simulink model "Preleva2"  (R2019a)
settings: Solver=VariableStepAuto  StartTime=0.0  StopTime=10.0  RelTol=1e-3
settings Model: Creator=anton  LastModifiedBy=anton

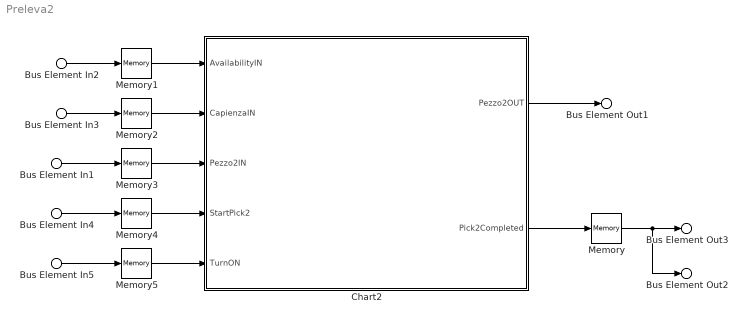
== system Preleva2 ==
  Bus Element In2 : Inport  PortName=Availability2IN
  Bus Element In3 : Inport  Port=2  PortName=Capienza2IN
  Bus Element In4 : Inport  Port=3  PortName=StartPick2
  Bus Element In5 : Inport  Port=4  PortName=TurnON
  Bus Element In1 : Inport  Port=5  PortName=Pezzo2
  Chart2 : Stateflow chart  BlockKeywords=__PRM__SERIALIZED__DATA__:Stateflow Chart,Stateflow Diagram  TreatAsAtomicUnit=on
  Memory{,1..5} (6 alike) : Memory
  Bus Element Out1 : Outport  PortName=Pezzo2OUT
  Bus Element Out2 : Outport  Port=2  PortName=Pick2Completed
  Bus Element Out3 : Outport  Port=3  PortName=Pick2CompletedOUT
  wires:
  Chart2/1(Pezzo2OUT) -> Bus Element Out1/1
  Chart2/2(Pick2Completed) -> Memory/1
  Memory/1 -> Bus Element Out2/1, Bus Element Out3/1
  Bus Element In5/1 -> Memory5/1
  Memory5/1 -> Chart2/5(TurnON)
  Bus Element In4/1 -> Memory4/1
  Memory4/1 -> Chart2/4(StartPick2)
  Bus Element In1/1 -> Memory3/1
  Memory3/1 -> Chart2/3(Pezzo2IN)
  Bus Element In2/1 -> Memory1/1
  Memory1/1 -> Chart2/1(AvailabilityIN)
  Bus Element In3/1 -> Memory2/1
  Memory2/1 -> Chart2/2(CapienzaIN)

== stateflow chart Preleva2/Chart2 ==
  state Idle
    Pezzo2OUT=0;
    Pick2Completed=0;
  state Waiting
    Pezzo2OUT=0;
    Pick2Completed=0;
  state Active
  state Working
  state Place
    during:
    Pezzo2OUT=1;
    Pick2Completed = 1;
    pause(0.1);
  state Pick
    pause(0.1);
  (default) -> Idle
  Idle -> Active : [TurnON==1]
  Place -> Idle [order 2] : [TurnON==0]
  Waiting -> Idle [order 2] : [TurnON==0]
  Pick -> Idle [order 2] : [TurnON==0]
  Working -> Idle [order 2] : [TurnON==0]
  Active -> Waiting
  Waiting -> Working [order 1] : [StartPick2==1]
  Place -> Waiting [order 1] : [after(1,sec)]
  Working -> Pick [order 1] : [AvailabilityIN==1 && CapienzaIN>0 && Pezzo2IN==1]
  Pick -> Place [order 1] : [after(10,sec)]
  data: AvailabilityIN input; CapienzaIN input; Pezzo2IN input; Pezzo2OUT output; StartPick2 input; Pick2Completed output; TurnON input
